simulink model "assignment2"  (R2017a)
settings: Solver=VariableStepAuto  StartTime=0.0  StopTime=50000  RelTol=1e-3
libraries: hdlsllib x3, simulink x1
settings Model: Creator=wachala.j  LastModifiedBy=wachala.j

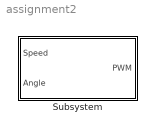
== system assignment2 ==
  Subsystem : Subsystem

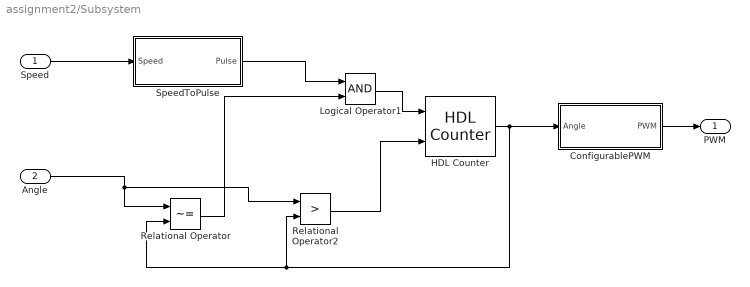
== system assignment2/Subsystem ==
  Speed : Inport
  Angle : Inport  Port=2
  ConfigurablePWM : Subsystem
  HDL Counter : hdlsllib/HDL Operations/HDL Counter  CountType=Count limited  CountInit=90  CountStep=1  CountMax=180  CountFromType=Initial value  CountFrom=90  CountResetPort=off  CountLoadPort=off  CountEnbPort=on  CountDirPort=on  CountDataType=Unsigned  CountWordLen=8  CountFracLen=0  CountSampTime=1
      settings: SourceProductName=HDL Coder  SourceProductBaseCode=HD
  Logical Operator1 : Logic  AllPortsSameDT=off  OutDataTypeStr=boolean
  Relational Operator : RelationalOperator  Operator=~=  OutDataTypeStr=boolean  RndMeth=Simplest
  Relational Operator2 : RelationalOperator  Operator=>  OutDataTypeStr=boolean  RndMeth=Simplest
  SpeedToPulse : Subsystem
  PWM : Outport
  wires:
  Relational Operator/1 -> Logical Operator1/2
  Relational Operator2/1 -> HDL Counter/2
  SpeedToPulse/1("Pulse ") -> Logical Operator1/1
  ConfigurablePWM/1(PWM) -> PWM/1
  Angle/1 -> Relational Operator2/1, Relational Operator/1
  Speed/1 -> SpeedToPulse/1(Speed)
  HDL Counter/1 -> ConfigurablePWM/1(Angle), Relational Operator2/2, Relational Operator/2
  Logical Operator1/1 -> HDL Counter/1

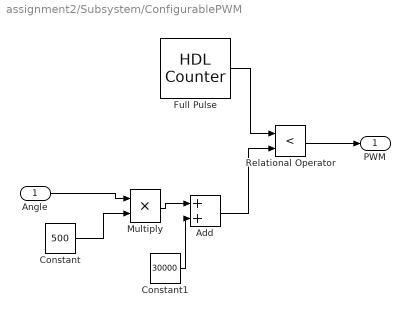
== system assignment2/Subsystem/ConfigurablePWM ==
  Angle : Inport  OutDataTypeStr=uint8
  Add : Sum
  Constant : Constant  Value=500  OutDataTypeStr=uint8
  Constant1 : Constant  Value=30000  OutDataTypeStr=uint8
  Full Pulse : hdlsllib/HDL Operations/HDL Counter  CountType=Count limited  CountInit=0  CountStep=1  CountMax=1000000  CountFromType=Initial value  CountFrom=0  CountResetPort=off  CountLoadPort=off  CountEnbPort=off  CountDirPort=off  CountDataType=Unsigned  CountWordLen=32  CountFracLen=0  CountSampTime=1
      settings: SourceProductName=HDL Coder  SourceProductBaseCode=HD
  Multiply : Product  Inputs=**
  Relational Operator : RelationalOperator  Operator=<  OutDataTypeStr=boolean  RndMeth=Simplest
  PWM : Outport
  wires:
  Relational Operator/1 -> PWM/1
  Full Pulse/1 -> Relational Operator/1
  Angle/1 -> Multiply/1
  Multiply/1 -> Add/1
  Constant1/1 -> Add/2
  Add/1 -> Relational Operator/2
  Constant/1 -> Multiply/2

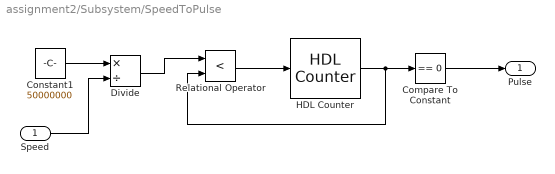
== system assignment2/Subsystem/SpeedToPulse ==
  Speed : Inport
  Compare To Constant : simulink/Logic and Bit Operations/Compare To Constant  relop===  const=0  OutDataTypeStr=boolean
  Constant1 : Constant  Value=50000000  SampleTime=1
  Divide : Product  Inputs=*/  SaturateOnIntegerOverflow=on  RndMeth=Zero
  HDL Counter : hdlsllib/HDL Operations/HDL Counter  CountType=Free running  CountInit=0  CountStep=1  CountMax=25  CountFromType=Initial value  CountFrom=0  CountResetPort=on  CountLoadPort=off  CountEnbPort=off  CountDirPort=off  CountDataType=Unsigned  CountWordLen=32  CountFracLen=0  CountSampTime=1
      settings: SourceProductName=HDL Coder  SourceProductBaseCode=HD
  Relational Operator : RelationalOperator  Operator=<  OutDataTypeStr=boolean  RndMeth=Simplest
  "Pulse " : Outport
  wires:
  HDL Counter/1 -> Relational Operator/2, Compare To Constant/1
  Divide/1 -> Relational Operator/1
  Relational Operator/1 -> HDL Counter/1
  Compare To Constant/1 -> "Pulse "/1
  Speed/1 -> Divide/2
  Constant1/1 -> Divide/1
